simulink model "phdMain"  (R2023b)
settings: Solver=ode4  StartTime=0.0  StopTime=t.Data(end)  FixedStep=1e-3  RelTol=1e-3
undefined symbols (not defined in the file): A_bar, AEFF, B_E, C_bar, C_T, Cd_neg, Cd_pos, DiscIntNeverNeededParam, Gamma, H, k, K, L_gain, L_STROKE, M, m3PsToLpm, P_return_Pa, P_supply_Pa, PA_Pa, PaToBar, PB_Pa, Q, R, RHO, Ts, V01, V02, V_DEAD, v_mPs, W, xc_dot, xc_m
libraries: simulink x1
(part 2 of 3)

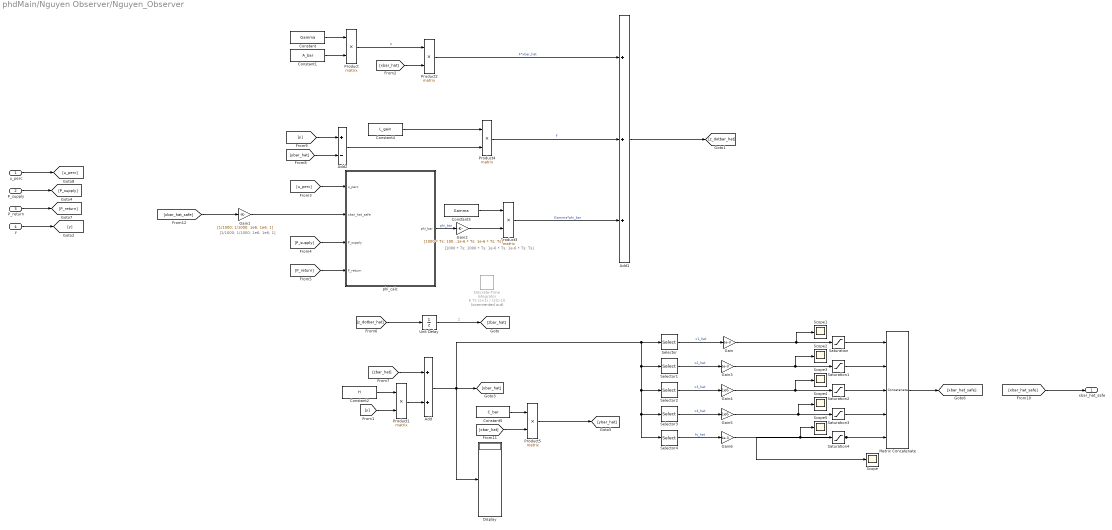
== system phdMain/Nguyen Observer/Nguyen_Observer ==
  note: [1000 * Ts; 1000 * Ts; 1e-6 * Ts; 1e-6 * Ts; Ts]
  note: [1/1000; 1/1000; 1e6; 1e6; 1]
  u_perc : Inport  PortDimensions=[1,1]
  P_supply : Inport  Port=2  OutDataTypeStr=double
  P_return : Inport  Port=3  OutDataTypeStr=double
  y : Inport  Port=4  PortDimensions=[4,1]
  Add : Sum
  Add1 : Sum  Inputs=+++
  Add2 : Sum  Inputs=+-
  Constant : Constant  Value=Gamma
  Constant1 : Constant  Value=A_bar
  Constant2 : Constant  Value=H
  Constant3 : Constant  Value=Gamma
  Constant4 : Constant  Value=L_gain
  Constant5 : Constant  Value=C_bar
  Discrete-Time Integrator : DiscreteIntegrator  Commented=on  IntegratorMethod=Integration: Trapezoidal  InitialCondition=[0,0,PA_Pa.Data(1)*1e-6,PB_Pa.Data(1)*1e-6,0]'  SampleTime=-1  ICPrevOutput=DiscIntNeverNeededParam  ICPrevScaledInput=DiscIntNeverNeededParam
  Display : Display
  Gain : Gain  Gain=1e-3
  Gain1 : Gain  Gain=[1/1000; 1/1000; 1e6; 1e6; 1]
  Gain2 : Gain  Gain=[1000 * Ts; 1000 * Ts; 1e-6 * Ts; 1e-6 * Ts; Ts]
  Gain3 : Gain  Gain=1e-3
  Gain4 : Gain  Gain=1e6
  Gain5 : Gain  Gain=1e6
  Gain6 : Gain  Gain=1e-3
  Matrix Concatenate : Concatenate  NumInputs=5  Mode=Multidimensional array
  Product{,1..5} (6 alike) : Product  Multiplication=Matrix(*)
  Saturation : Saturate  UpperLimit=L_STROKE  LowerLimit=-L_STROKE
  Saturation1 : Saturate  UpperLimit=2  LowerLimit=-2
  Saturation2 : Saturate  UpperLimit=200e5  LowerLimit=4e5
  Saturation3 : Saturate  UpperLimit=200e5  LowerLimit=4e5
  Saturation4 : Saturate  UpperLimit=L_STROKE  LowerLimit=-L_STROKE
  Scope{,1..5} (6 alike) : Scope
  Selector : Selector  InputPortWidth=5  IndexOptions=Index vector (dialog)  Indices=1  OutputSizes=1
  Selector1 : Selector  InputPortWidth=5  IndexOptions=Index vector (dialog)  Indices=2  OutputSizes=1
  Selector2 : Selector  InputPortWidth=5  IndexOptions=Index vector (dialog)  Indices=3  OutputSizes=1
  Selector3 : Selector  InputPortWidth=5  IndexOptions=Index vector (dialog)  Indices=4  OutputSizes=1
  Selector4 : Selector  InputPortWidth=5  IndexOptions=Index vector (dialog)  Indices=5  OutputSizes=1
  Unit Delay : UnitDelay  InitialCondition=[0,0,PA_Pa.Data(1)*1e-6,PB_Pa.Data(1)*1e-6,0]'  SampleTime=Ts  HasFrameUpgradeWarning=on
  phi_calc : Subsystem
  xbar_hat_safe : Outport
  wires:
  [y] -> Add2/1
  Product3/1 -> Add1/3  "Gamma*phi_bar"
  [u_perc] -> phi_calc/1(u_perc)
  Add2/1 -> Product4/2
  u_perc/1 -> [u_perc]
  Constant3/1 -> Product3/1
  Unit Delay/1 -> [zbar_hat]  "z"
  [ybar_hat] -> Add2/2
  Constant2/1 -> Product1/1
  Product/1 -> Product2/1  "F"
  [P_return] -> phi_calc/4(P_return)
  Constant1/1 -> Product/2
  Product2/1 -> Add1/1  "F*xbar_hat"
  Constant/1 -> Product/1
  [xbar_hat] -> Product2/2
  P_return/1 -> [P_return]
  [y] -> Product1/2
  [zbar_hat] -> Add/1
  y/1 -> [y]
  Add1/1 -> [z_dotbar_hat]
  Product4/1 -> Add1/2  "F"
  Product1/1 -> Add/2
  P_supply/1 -> [P_supply]
  phi_calc/1(phi_bar) -> Gain2/1  "phi_bar"
  [P_supply] -> phi_calc/3(P_supply)
  [z_dotbar_hat] -> Unit Delay/1
  [xbar_hat_safe] -> xbar_hat_safe/1
  Constant5/1 -> Product5/1
  [xbar_hat] -> Product5/2
  Product5/1 -> [ybar_hat]
  Selector3/1 -> Gain5/1  "x4_hat"
  Selector2/1 -> Gain4/1  "x3_hat"
  Selector1/1 -> Gain3/1  "x2_hat"
  Saturation/1 -> Matrix Concatenate/1
  Saturation1/1 -> Matrix Concatenate/2
  Saturation2/1 -> Matrix Concatenate/3
  Saturation3/1 -> Matrix Concatenate/4
  Saturation4/1 -> Scope/1, Matrix Concatenate/5
  Matrix Concatenate/1 -> [xbar_hat_safe]
  Selector4/1 -> Gain6/1  "fs_hat"
  Selector/1 -> Gain/1  "x1_hat"
  Constant4/1 -> Product4/1
  Add/1 -> Selector3/1, Selector4/1, Selector2/1, Selector1/1, Selector/1, [xbar_hat], Display/1
  [xbar_hat_safe] -> Gain1/1
  Gain1/1 -> phi_calc/2(xbar_hat_safe)
  Gain2/1 -> Product3/2
  Gain/1 -> Scope1/1, Saturation/1
  Gain3/1 -> Scope2/1, Saturation1/1
  Gain4/1 -> Saturation2/1, Scope3/1
  Gain5/1 -> Saturation3/1, Scope4/1
  Gain6/1 -> Scope5/1, Saturation4/1

== system phdMain/Reference_Generator/Sine_Generator ==
  Amp_mm : Inport  OutDataTypeStr=double
  f_Hz : Inport  Port=2
  phi_deg : Inport  Port=3  OutDataTypeStr=double
  Add : Sum
  Clock : Clock
  Constant : Constant  Value=2
  Constant1 : Constant  Value=3.14159265359
  Constant2 : Constant  Value=3.14159265359
  Constant3 : Constant  Value=180
  Constant4 : Constant  Value=1e-3
  Math Reciprocal : Math  Operator=reciprocal  SignedPower=on
  Product : Product  Inputs=4
  Product{1..4} (4 alike) : Product
  Sin : Trigonometry
  r : Outport
  wires:
  Constant1/1 -> Product/2
  Constant/1 -> Product/1
  f_Hz/1 -> Product/3
  phi_deg/1 -> Product1/1
  Constant2/1 -> Product2/1
  Constant3/1 -> Math Reciprocal/1
  Math Reciprocal/1 -> Product2/2
  Product2/1 -> Product1/2
  Clock/1 -> Product/4
  Product/1 -> Sin/1
  Sin/1 -> Product3/2
  Product1/1 -> Add/2
  Product3/1 -> Add/1
  Add/1 -> r/1
  Amp_mm/1 -> Product4/2
  Product4/1 -> Product3/1
  Constant4/1 -> Product4/1

== system phdMain/Reverse_PressureModel/Q_returnleak ==
  Add : Sum  Inputs=+-
  Constant5 : Constant  Value=70e5
  Divide : Product  Inputs=*/
  From Workspace20 : FromWorkspace  VariableName=P_supply_Pa
  From Workspace21 : FromWorkspace  VariableName=P_return_Pa
  Gain2 : Gain  Gain=0.53
  Sqrt : Sqrt
  Out1 : Outport
  wires:
  Constant5/1 -> Divide/2
  From Workspace20/1 -> Add/1  "P_supply"
  From Workspace21/1 -> Add/2  "P_return"
  Gain2/1 -> Out1/1
  Add/1 -> Divide/1
  Sqrt/1 -> Gain2/1
  Divide/1 -> Sqrt/1

== system phdMain/Reverse_PressureModel1/Q_returnleak ==
  Add : Sum  Inputs=+-
  Constant5 : Constant  Value=70e5
  Divide : Product  Inputs=*/
  From Workspace20 : FromWorkspace  VariableName=P_supply_Pa
  From Workspace21 : FromWorkspace  VariableName=P_return_Pa
  Gain2 : Gain  Gain=0.53
  Sqrt : Sqrt
  Out1 : Outport
  wires:
  Divide/1 -> Sqrt/1
  Sqrt/1 -> Gain2/1
  Add/1 -> Divide/1
  Gain2/1 -> Out1/1
  From Workspace21/1 -> Add/2  "P_return"
  From Workspace20/1 -> Add/1  "P_supply"
  Constant5/1 -> Divide/2

== system phdMain/SDRE_OBS_SNR/Subsystem ==
  Constant3 : Constant  Value=[1 0 0 0;0 0 1 0; 0 0 0 1]
  Constant4 : Constant  Value=mean(P_return_Pa)
  Constant5 : Constant  Value=Q
  Constant6 : Constant  Value=mean(P_supply_Pa)
  Constant7 : Constant  Value=R
  Discrete Algebraic Riccati Eqn : Subsystem
  MATLAB Function : MATLAB Function  TreatAsAtomicUnit=on
  MATLAB Function1 : MATLAB Function  TreatAsAtomicUnit=on
  MATLAB Function2 : MATLAB Function  TreatAsAtomicUnit=on
  Terminator : Terminator
  wires:
  [x4_hat] -> MATLAB Function2/5(x4_hat)
  MATLAB Function2/1(Q1) -> MATLAB Function1/1(Q1_calc)
  [x3_hat] -> MATLAB Function2/4(x3_hat)
  MATLAB Function1/1(B_x) -> Discrete Algebraic Riccati Eqn/2(B_k)
  [x1_hat] -> MATLAB Function/1(x_1_hat)
  Constant4/1 -> MATLAB Function2/3(Pr)
  MATLAB Function2/3(QR) -> Terminator/1
  MATLAB Function2/2(Q2) -> MATLAB Function1/2(Q2_calc)
  ? -> MATLAB Function2/1(u)
  [x2_hat] -> MATLAB Function/2(x_2_hat)
  Constant6/1 -> MATLAB Function2/2(Ps)
  Constant3/1 -> Discrete Algebraic Riccati Eqn/4(H)
  [y] -> Discrete Algebraic Riccati Eqn/3(y)
  Constant7/1 -> Discrete Algebraic Riccati Eqn/6(R)
  Constant5/1 -> Discrete Algebraic Riccati Eqn/5(Q)
  MATLAB Function/1(A_x) -> Discrete Algebraic Riccati Eqn/1(A_k)

== system phdMain/Subsystem3/Subsystem ==
  y : Inport
  phi2_hat : Inport  Port=2
  d1_hat : Inport  Port=3
  l1 : Inport  Port=4
  eta : Inport  Port=5
  phi1_hat : Inport  Port=6
  Add : Sum  Inputs=+-
  Add1 : Sum
  Add2 : Sum
  Product : Product
  Product1 : Product
  phi1_hat_dot : Outport
  wires:
  eta/1 -> Product/2
  l1/1 -> Product/1
  phi1_hat/1 -> Add/2
  y/1 -> Add/1
  Product/1 -> Product1/1
  Add/1 -> Product1/2
  Product1/1 -> Add1/2
  d1_hat/1 -> Add1/1
  Add1/1 -> Add2/2
  phi2_hat/1 -> Add2/1
  Add2/1 -> phi1_hat_dot/1

== system phdMain/Subsystem3/Subsystem1 ==
  phi1_hat : Inport
  d2_hat : Inport  Port=2
  l2 : Inport  Port=3
  eta : Inport  Port=4
  y : Inport  Port=5
  x3 : Inport  Port=6
  x4 : Inport  Port=7
  phi2_hat : Inport  Port=8
  Add : Sum  Inputs=+-
  Add1 : Sum
  Add2 : Sum
  Add3 : Sum  Inputs=+++
  Constant : Constant  Value=AEFF
  Constant1 : Constant  Value=M
  Divide : Product  Inputs=*/  RndMeth=Zero  SaturateOnIntegerOverflow=on
  Gain : Gain  Gain=1/M
  Lugre_Model : Subsystem
  Product{,1,3..4} (4 alike) : Product
  Unary Minus1 : UnaryMinus
  phi2_hat_dot : Outport
  wires:
  Add2/1 -> phi2_hat_dot/1
  Add1/1 -> Add2/2
  d2_hat/1 -> Add1/1
  Product1/1 -> Add1/2
  Add/1 -> Product1/2
  Product/1 -> Product1/1
  y/1 -> Add/1
  phi1_hat/1 -> Add/2
  l2/1 -> Product/1
  eta/1 -> Product/2
  Divide/1 -> Product3/1, Unary Minus1/1  "a23"
  x3/1 -> Product3/2
  Unary Minus1/1 -> Product4/1  "a24"
  x4/1 -> Product4/2
  Product3/1 -> Add3/2
  Product4/1 -> Add3/3
  Add3/1 -> Add2/1
  phi2_hat/1 -> Lugre_Model/1(xc_dot)
  Gain/1 -> Add3/1
  Lugre_Model/1(F_friction) -> Gain/1  "F_friction"
  Constant/1 -> Divide/1
  Constant1/1 -> Divide/2

== system phdMain/Subsystem3/Subsystem3 ==
  phi2_hat : Inport
  gamma1 : Inport  Port=2
  phi1_hat : Inport  Port=3
  sigma1_hat : Inport  Port=4
  Add : Sum
  Add1 : Sum
  Product : Product
  Product1 : Product
  Unary Minus : UnaryMinus
  sigma1_hat_dot : Outport
  wires:
  sigma1_hat/1 -> Add/1
  Product/1 -> Add/2
  Add/1 -> Add1/2
  phi2_hat/1 -> Add1/1
  gamma1/1 -> Unary Minus/1, Product/2
  phi1_hat/1 -> Product/1
  Add1/1 -> Product1/1
  Unary Minus/1 -> Product1/2
  Product1/1 -> sigma1_hat_dot/1

== system phdMain/Subsystem3/Subsystem4 ==
  phi2_hat : Inport
  gamma2 : Inport  Port=2
  x3 : Inport  Port=3
  x4 : Inport  Port=4
  sigma2_hat : Inport  Port=5
  Add : Sum
  Add2 : Sum
  Add3 : Sum  Inputs=+++
  Constant : Constant  Value=AEFF
  Constant1 : Constant  Value=M
  Divide : Product  Inputs=*/  RndMeth=Zero  SaturateOnIntegerOverflow=on
  Gain : Gain  Gain=1/M
  Lugre_Model : Subsystem
  Product{,1,3..4} (4 alike) : Product
  Unary Minus : UnaryMinus
  Unary Minus1 : UnaryMinus
  sigma2_hat_dot : Outport
  wires:
  Product1/1 -> sigma2_hat_dot/1
  gamma2/1 -> Unary Minus/1, Product/2
  Product/1 -> Add/2
  sigma2_hat/1 -> Add/1
  Product3/1 -> Add3/2
  Product4/1 -> Add3/3
  x4/1 -> Product4/2
  phi2_hat/1 -> Product/1, Lugre_Model/1(xc_dot)
  Unary Minus1/1 -> Product4/1  "a24"
  x3/1 -> Product3/2
  Add3/1 -> Add2/1
  Gain/1 -> Add3/1
  Add/1 -> Add2/2
  Add2/1 -> Product1/1
  Unary Minus/1 -> Product1/2
  Lugre_Model/1(F_friction) -> Gain/1  "F_friction"
  Constant/1 -> Divide/1
  Divide/1 -> Product3/1, Unary Minus1/1  "a23"
  Constant1/1 -> Divide/2

== system phdMain/Subsystem3/Subsystem6 ==
  sigma1_hat : Inport
  gamma1 : Inport  Port=2
  phi1_hat : Inport  Port=3
  Add : Sum
  Product : Product
  d1_hat : Outport
  wires:
  sigma1_hat/1 -> Add/1
  gamma1/1 -> Product/1
  phi1_hat/1 -> Product/2
  Product/1 -> Add/2
  Add/1 -> d1_hat/1

== system phdMain/Subsystem3/Subsystem7 ==
  sigma2_hat : Inport
  gamma2 : Inport  Port=2
  phi2_hat : Inport  Port=3
  Add : Sum
  Product : Product
  d2_hat : Outport
  wires:
  gamma2/1 -> Product/1
  sigma2_hat/1 -> Add/1
  Product/1 -> Add/2
  Add/1 -> d2_hat/1
  phi2_hat/1 -> Product/2

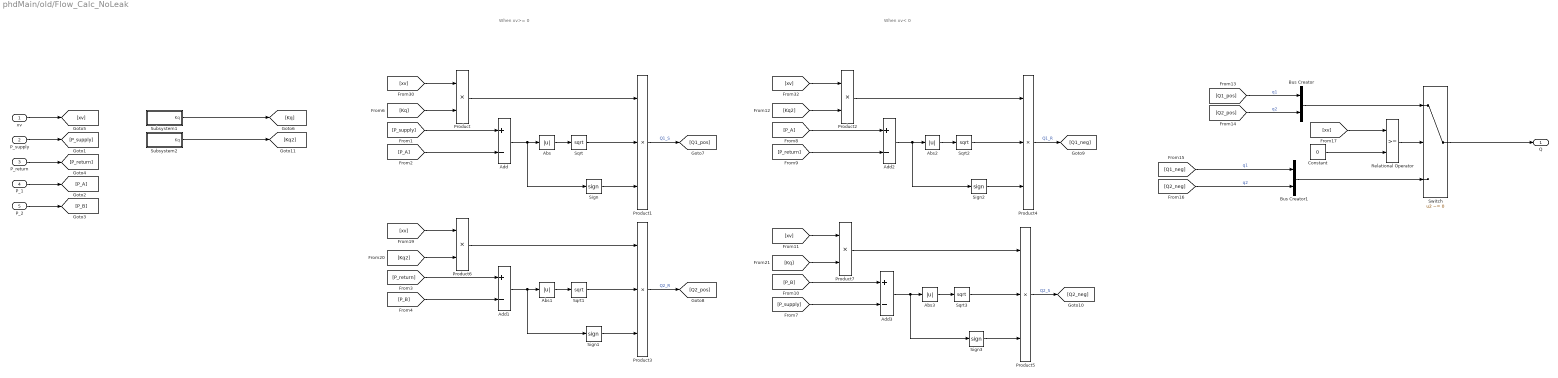
== system phdMain/old/Flow_Calc_NoLeak ==
  note: When xv< 0
  note: When xv>= 0
  xv : Inport  OutDataTypeStr=double
  P_supply : Inport  Port=2  OutDataTypeStr=double
  P_return : Inport  Port=3  OutDataTypeStr=double
  P_1 : Inport  Port=4  OutDataTypeStr=double
  P_2 : Inport  Port=5  OutDataTypeStr=double
  Abs{,1..3} (4 alike) : Abs  SaturateOnIntegerOverflow=off
  Add{,1..3} (4 alike) : Sum  Inputs=+-
  Bus Creator : BusCreator  Inputs=2
  Bus Creator1 : BusCreator  Inputs=2
  Constant : Constant  Value=0  OutDataTypeStr=double
  Product{,2,6..7} (4 alike) : Product
  Product{1,3..5} (4 alike) : Product  Inputs=3
  Relational Operator : RelationalOperator  OutDataTypeStr=boolean  RndMeth=Simplest  InputSameDT=off
  Sign{,1..3} (4 alike) : Signum
  Sqrt{,1..3} (4 alike) : Sqrt
  Subsystem1 : Subsystem
  Subsystem2 : Subsystem
  Switch : Switch  Criteria=u2 ~= 0  SaturateOnIntegerOverflow=off  InputSameDT=off
  Q : Outport  OutDataTypeStr=double
  wires:
  Subsystem2/1(Kq) -> [Kq2]
  Subsystem1/1(Kq) -> [Kq]
  Product5/1 -> [Q2_neg]  "Q2_S"
  Product4/1 -> [Q1_neg]  "Q1_R"
  Product3/1 -> [Q2_pos]  "Q2_R"
  Product1/1 -> [Q1_pos]  "Q1_S"
  Switch/1 -> Q/1
  [xv] -> Product/1
  [Q1_neg] -> Bus Creator1/1  "q1"
  [Q2_pos] -> Bus Creator/2  "q2"
  Product7/1 -> Product5/1
  [xv] -> Product7/1
  [Kq] -> Product7/2
  Product6/1 -> Product3/1
  [Kq2] -> Product6/2
  [xv] -> Product6/1
  Bus Creator1/1 -> Switch/3
  Bus Creator/1 -> Switch/1
  Relational Operator/1 -> Switch/2
  Constant/1 -> Relational Operator/2
  [xv] -> Relational Operator/1
  [Q2_neg] -> Bus Creator1/2  "q2"
  [Q1_pos] -> Bus Creator/1  "q1"
  [P_supply] -> Add3/2
  [P_B] -> Add3/1
  [P_return] -> Add2/2
  [P_A] -> Add2/1
  Product2/1 -> Product4/1
  Sqrt2/1 -> Product4/2
  Abs2/1 -> Sqrt2/1
  Add2/1 -> Abs2/1, Sign2/1
  Sign2/1 -> Product4/3
  Sign3/1 -> Product5/3
  Add3/1 -> Sign3/1, Abs3/1
  Abs3/1 -> Sqrt3/1
  Sqrt3/1 -> Product5/2
  [Kq2] -> Product2/2
  [xv] -> Product2/1
  xv/1 -> [xv]
  P_return/1 -> [P_return]
  P_2/1 -> [P_B]
  P_1/1 -> [P_A]
  P_supply/1 -> [P_supply]
  [P_B] -> Add1/2
  [P_return] -> Add1/1
  [Kq] -> Product/2
  Sqrt1/1 -> Product3/2
  Abs1/1 -> Sqrt1/1
  Add1/1 -> Abs1/1, Sign1/1
  Sign1/1 -> Product3/3
  Sign/1 -> Product1/3
  Add/1 -> Sign/1, Abs/1
  Abs/1 -> Sqrt/1
  Sqrt/1 -> Product1/2
  Product/1 -> Product1/1
  [P_A] -> Add/2
  [P_supply] -> Add/1

== system phdMain/old/Flow_Calc_WithLeak ==
  xv : Inport  OutDataTypeStr=double
  P_supply : Inport  Port=2  OutDataTypeStr=double
  P_return : Inport  Port=3  OutDataTypeStr=double
  P_1 : Inport  Port=4  OutDataTypeStr=double
  P_2 : Inport  Port=5  OutDataTypeStr=double
  Bus Creator4 : BusCreator  Inputs=2
  Constant1 : Constant  Value=RHO
  Constant19 : Constant  Value=3e-6
  Constant20 : Constant  Value=4e-6
  Constant22 : Constant  Value=0.6240657450358073
  Constant23 : Constant  Value=0.1382171870867411
  Constant24 : Constant  Value=0.7
  Constant26 : Constant  Value=82.43058647155762
  Constant27 : Constant  Value=W
  Constant28 : Constant  Value=0.01
  From Workspace2 : FromWorkspace  VariableName=[t.t, t.Q_return_m3Ps]
  Gain7 : Gain  Gain=m3PsToLpm
  Gain8 : Gain  Gain=1e-5
  Knob : KnobBlock  ScaleMin=0.1  ScaleMax=2
  Knob1 : KnobBlock  ScaleMin=0.1
  Knob2 : KnobBlock  ScaleMin=0.1  ScaleMax=2
  MATLAB Function2 : MATLAB Function  TreatAsAtomicUnit=on
  ReturnFlowDynamics1 : TransferFcn  Numerator=[28.61 633.5]  Denominator=[1 12.94 274.5 817.1]
  Scope : Scope  NumInputPorts=3
  q_withLeaks : Outport  OutDataTypeStr=double
  wires:
  P_supply/1 -> [P_supply]
  P_1/1 -> [P_A]
  P_2/1 -> [P_B]
  P_return/1 -> [P_return]
  xv/1 -> [xv]
  [xv] -> MATLAB Function2/1(xv)
  [P_supply] -> MATLAB Function2/2(P_P)
  [P_return] -> MATLAB Function2/3(P_T), MATLAB Function2/4(P_R)
  [P_A] -> MATLAB Function2/5(P_A)
  [P_B] -> MATLAB Function2/6(P_B)
  Constant27/1 -> MATLAB Function2/7(w)  "w"
  Constant19/1 -> MATLAB Function2/8(c)  "c"
  Constant20/1 -> MATLAB Function2/9(r)  "r"
  Constant1/1 -> MATLAB Function2/10(rho)  "rho"
  Constant28/1 -> MATLAB Function2/11(mu)  "mu"
  Constant24/1 -> MATLAB Function2/12(Cd)  "Cd"
  Constant22/1 -> MATLAB Function2/13(bias_P_dynamic)  "bias_P_dynamic"
  Constant23/1 -> MATLAB Function2/14(bias_T_dynamic)  "bias_T_dynamic"
  From Workspace2/1 -> Gain7/1
  Bus Creator4/1 -> q_withLeaks/1
  MATLAB Function2/1(Q_A) -> Bus Creator4/1  "q1"
  MATLAB Function2/2(Q_B) -> Bus Creator4/2  "q2"
  Constant26/1 -> Gain8/1  "x_leak"
  Gain8/1 -> MATLAB Function2/15(x_leak)
  MATLAB Function2/4(Q_return_model_lpm) -> [Q_return_model_lpm]
  MATLAB Function2/3(Q_Leak_Total_lpm) -> [Q_Leak_Total_lpm]
  Gain7/1 -> Scope/1  "Q_return_lpm"
  ReturnFlowDynamics1/1 -> Scope/3  "Q_returnTF_lpm"
  [Q_return_model_lpm] -> ReturnFlowDynamics1/1, Scope/2  "Q_return_model_lpm"

== system phdMain/old/ServoValve_Dynamics ==
  note: Deadband
  u : Inport  OutDataTypeStr=double
  Convert_SpoolPosition : Subsystem
  Dead Zone : DeadZone  LowerValue=-0.05  UpperValue=0.05
  Subsystem : Subsystem  Commented=on
  Valve Dynamics : TransferFcn  Numerator=[2.0884e+06]  Denominator=[1 2*1*1.4451e+03 2.0884e+06]
  xv : Outport  OutDataTypeStr=double
  wires:
  Dead Zone/1 -> Valve Dynamics/1
  u/1 -> Dead Zone/1
  Convert_SpoolPosition/1(xv) -> xv/1
  Valve Dynamics/1 -> Convert_SpoolPosition/1(u_perc)

== system phdMain/Cylinder_Dynamics/Lugre_Model/Subsystem1 ==
  term : Inport
  z_prev : Inport  Port=2
  v : Inport  Port=3
  Add : Sum
  Add1 : Sum
  Constant : Constant
  Gain : Gain  Gain=1e-3
  Gain1 : Gain  Gain=1e-3
  Math Reciprocal2 : Math  Operator=reciprocal  SignedPower=on
  Product : Product
  z : Outport
  wires:
  term/1 -> Gain1/1
  z_prev/1 -> Add/1
  v/1 -> Gain/1
  Gain/1 -> Add/2
  Add/1 -> Product/1
  Gain1/1 -> Add1/2
  Constant/1 -> Add1/1
  Add1/1 -> Math Reciprocal2/1
  Math Reciprocal2/1 -> Product/2
  Product/1 -> z/1

== system phdMain/Cylinder_Dynamics/Subsystem/Subsystem ==
  v_est : Inport
  MATLAB Function : MATLAB Function  TreatAsAtomicUnit=on
  F_statik : Outport
  wires:
  v_est/1 -> MATLAB Function/1(v)
  MATLAB Function/1(F_statik) -> F_statik/1

== system phdMain/Cylinder_Dynamics/Subsystem/Subsystem1 ==
  v_est : Inport
  MATLAB Function : MATLAB Function  TreatAsAtomicUnit=on
  F_statik : Outport
  wires:
  MATLAB Function/1(F_statik) -> F_statik/1
  v_est/1 -> MATLAB Function/1(v)

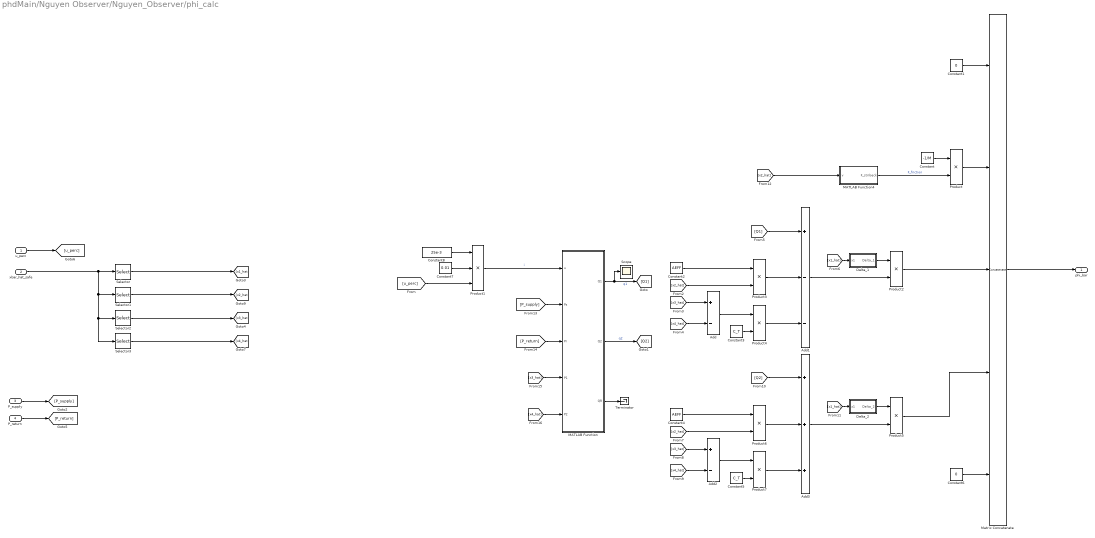
== system phdMain/Nguyen Observer/Nguyen_Observer/phi_calc ==
  u_perc : Inport
  xbar_hat_safe : Inport  Port=2
  P_supply : Inport  Port=3  OutDataTypeStr=double
  P_return : Inport  Port=4  OutDataTypeStr=double
  Add : Sum  Inputs=+-
  Add1 : Sum  Inputs=+--
  Add2 : Sum  Inputs=+-
  Add3 : Sum  Inputs=+++
  Constant : Constant  Value=-1/M
  Constant1 : Constant  Value=0
  Constant2 : Constant  Value=AEFF
  Constant3 : Constant  Value=C_T
  Constant4 : Constant  Value=AEFF
  Constant5 : Constant  Value=C_T
  Constant6 : Constant  Value=0
  Constant7 : Constant  Value=0.01
  Constant8 : Constant  Value=25e-3
  Delta_1 : Subsystem
  Delta_2 : Subsystem
  MATLAB Function : MATLAB Function  TreatAsAtomicUnit=on
  MATLAB Function4 : MATLAB Function  TreatAsAtomicUnit=on
  Matrix Concatenate : Concatenate  NumInputs=5  Mode=Multidimensional array
  Product{,2..7} (7 alike) : Product
  Product1 : Product  Inputs=3
  Scope : Scope
  Selector : Selector  InputPortWidth=5  IndexOptions=Index vector (dialog)  Indices=1  OutputSizes=1
  Selector1 : Selector  InputPortWidth=5  IndexOptions=Index vector (dialog)  Indices=2  OutputSizes=1
  Selector2 : Selector  InputPortWidth=5  IndexOptions=Index vector (dialog)  Indices=3  OutputSizes=1
  Selector3 : Selector  InputPortWidth=5  IndexOptions=Index vector (dialog)  Indices=4  OutputSizes=1
  Terminator : Terminator
  phi_bar : Outport
  wires:
  MATLAB Function4/1(F_stribeck) -> Product/2  "F_friction"
  Constant/1 -> Product/1
  MATLAB Function/1(Q1) -> Scope/1, [Q1]  "q1"
  MATLAB Function/2(Q2) -> [Q2]  "q2"
  [Q1] -> Add1/1
  [x2_hat] -> Product3/2
  [x4_hat] -> Add/2
  [x3_hat] -> Add/1
  Add/1 -> Product4/1
  Constant3/1 -> Product4/2
  Product3/1 -> Add1/2
  Product4/1 -> Add1/3
  Add1/1 -> Product2/2
  Delta_1/1(Delta_1) -> Product2/1
  [x1_hat] -> Delta_1/1(x1)
  [x1_hat] -> Delta_2/1(x1)
  Delta_2/1(Delta_2) -> Product5/1
  Add3/1 -> Product5/2
  Product7/1 -> Add3/3
  Product6/1 -> Add3/2
  Constant5/1 -> Product7/2
  Add2/1 -> Product7/1
  [x3_hat] -> Add2/1
  [x4_hat] -> Add2/2
  [x2_hat] -> Product6/2
  [Q2] -> Add3/1
  Constant6/1 -> Matrix Concatenate/5
  Product5/1 -> Matrix Concatenate/4
  Product/1 -> Matrix Concatenate/2
  Constant1/1 -> Matrix Concatenate/1
  Constant7/1 -> Product1/2
  Constant8/1 -> Product1/1
  Product1/1 -> MATLAB Function/1(u)  "i"
  u_perc/1 -> [u_perc]
  P_return/1 -> [P_return]
  P_supply/1 -> [P_supply]
  [u_perc] -> Product1/3
  [P_supply] -> MATLAB Function/2(Ps)
  [P_return] -> MATLAB Function/3(Pr)
  [x3_hat] -> MATLAB Function/4(P1)
  [x4_hat] -> MATLAB Function/5(P2)
  MATLAB Function/3(QR) -> Terminator/1
  Matrix Concatenate/1 -> phi_bar/1
  Selector/1 -> [x1_hat]
  Selector1/1 -> [x2_hat]
  Selector2/1 -> [x3_hat]
  Selector3/1 -> [x4_hat]
  Constant2/1 -> Product3/1
  Constant4/1 -> Product6/1
  Product2/1 -> Matrix Concatenate/3
  [x2_hat] -> MATLAB Function4/1(v)
  xbar_hat_safe/1 -> Selector3/1, Selector2/1, Selector1/1, Selector/1

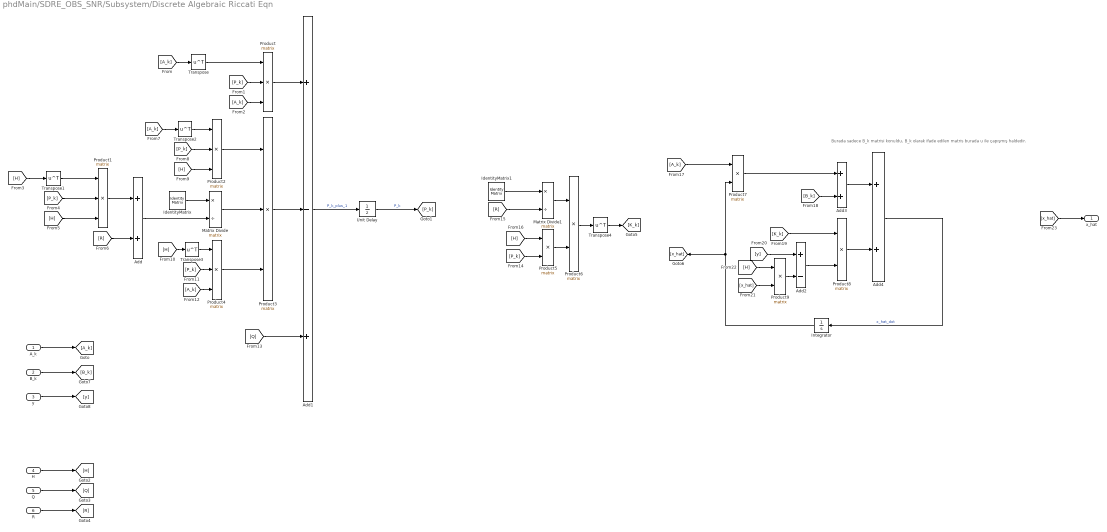
== system phdMain/SDRE_OBS_SNR/Subsystem/Discrete Algebraic Riccati Eqn ==
  note: Burada sadece B_k matrisi konuldu, B_k olarak ifade edilen matris burada u ile çapışmış haldedir.
  A_k : Inport  PortDimensions=[4,4]
  B_k : Inport  Port=2  PortDimensions=[4,1]
  y : Inport  Port=3
  H : Inport  Port=4
  Q : Inport  Port=5
  R : Inport  Port=6
  Add : Sum
  Add1 : Sum  Inputs=+-+
  Add2 : Sum  Inputs=+-
  Add3 : Sum
  Add4 : Sum
  IdentityMatrix : IdentityMatrix  OutputDimensions=4  SampleTime=1e-3
  IdentityMatrix1 : IdentityMatrix  OutputDimensions=3  SampleTime=1e-3
  Integrator : Integrator
  Matrix Divide : Product  Inputs=*/  Multiplication=Matrix(*)
  Matrix Divide1 : Product  Inputs=*/  Multiplication=Matrix(*)
  Product{,1..4} (5 alike) : Product  Inputs=3  Multiplication=Matrix(*)
  Product{5..9} (5 alike) : Product  Multiplication=Matrix(*)
  Transpose{,1..4} (5 alike) : Math  Operator=transpose
  Unit Delay : UnitDelay  SampleTime=-1  HasFrameUpgradeWarning=on
  x_hat : Outport
  wires:
  A_k/1 -> [A_k]
  [A_k] -> Transpose/1
  Transpose/1 -> Product/1
  [P_k] -> Product/2
  [A_k] -> Product/3
  H/1 -> [H]
  IdentityMatrix/1 -> Matrix Divide/1
  [H] -> Transpose1/1
  Transpose1/1 -> Product1/1
  [P_k] -> Product1/2
  [H] -> Product1/3
  Product1/1 -> Add/1
  [R] -> Add/2
  Add/1 -> Matrix Divide/2
  [A_k] -> Transpose2/1
  Transpose2/1 -> Product2/1
  [P_k] -> Product2/2
  [H] -> Product2/3
  Product2/1 -> Product3/1
  [P_k] -> Product4/2
  [H] -> Transpose3/1
  Transpose3/1 -> Product4/1
  [A_k] -> Product4/3
  Matrix Divide/1 -> Product3/2
  Product4/1 -> Product3/3
  Product/1 -> Add1/1
  Product3/1 -> Add1/2
  [Q] -> Add1/3
  Add1/1 -> Unit Delay/1  "P_k_plus_1"
  Unit Delay/1 -> [P_k]  "P_k"
  Q/1 -> [Q]
  R/1 -> [R]
  Matrix Divide1/1 -> Product6/1
  [R] -> Matrix Divide1/2
  IdentityMatrix1/1 -> Matrix Divide1/1
  [P_k] -> Product5/2
  [H] -> Product5/1
  Product5/1 -> Product6/2
  Product6/1 -> Transpose4/1
  Transpose4/1 -> [K_k]
  [A_k] -> Product7/1
  Integrator/1 -> [x_hat], Product7/2
  Product7/1 -> Add3/1
  [B_k] -> Add3/2
  B_k/1 -> [B_k]
  [K_k] -> Product8/1
  y/1 -> [y]
  [y] -> Add2/1
  Product9/1 -> Add2/2
  [x_hat] -> Product9/2
  [H] -> Product9/1
  Add2/1 -> Product8/2
  Product8/1 -> Add4/2
  Add3/1 -> Add4/1
  Add4/1 -> Integrator/1  "x_hat_dot"
  [x_hat] -> x_hat/1

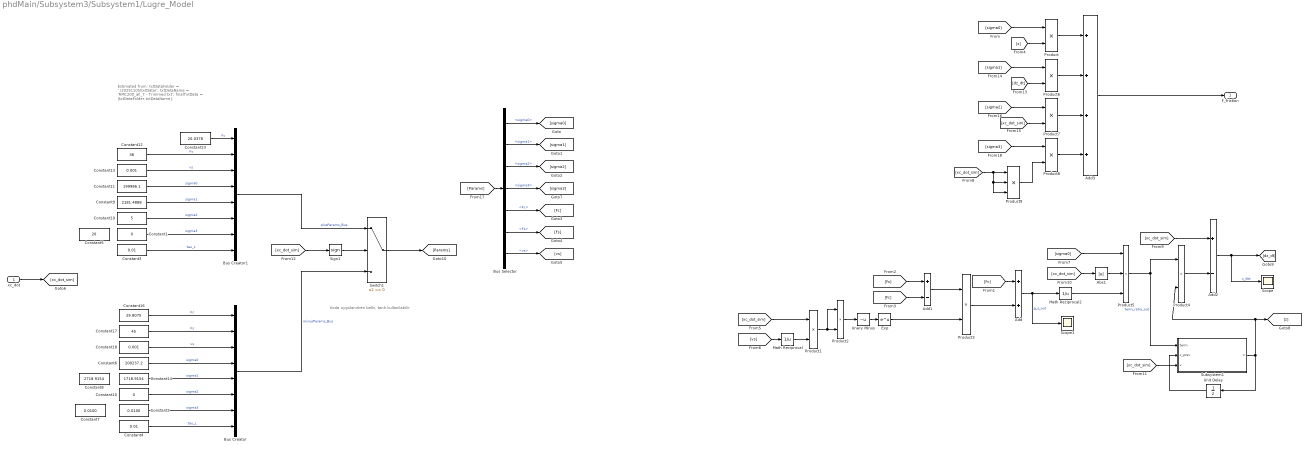
== system phdMain/Subsystem3/Subsystem1/Lugre_Model ==
  note: Koda uygulanırken belki, tanh kullanılabilir
  note: Estimated from:
      |
      | txtDataFolder = '.\20251105\txtData\';
      | txtDataName = 'RMC200_all_7 - Trimmed.txt';
      | finalTxtData = [txtDataFolder,txtDataName];
  xc_dot : Inport  OutDataTypeStr=double
  Abs1 : Abs  SaturateOnIntegerOverflow=off
  Add : Sum
  Add1 : Sum  Inputs=+-
  Add2 : Sum  Inputs=+-
  Add3 : Sum  Inputs=++++
  Bus Selector : BusSelector  OutputSignals=sigma0,sigma1,sigma2,sigma3,Fc,Fs,vs
  Bus Creator : BusCreator  Inputs=8
  Bus Creator1 : BusCreator  Inputs=8
  Constant1 : Constant  Value=0  OutDataTypeStr=double
  Constant10 : Constant  Value=0  OutDataTypeStr=double
  Constant11 : Constant  Value=199986.1  OutDataTypeStr=double
  Constant12 : Constant  Value=38  OutDataTypeStr=double
  Constant13 : Constant  Value=0.001  OutDataTypeStr=double
  Constant14 : Constant  Value=1718.9154  OutDataTypeStr=double
  Constant16 : Constant  Value=29.8075  OutDataTypeStr=double
  Constant17 : Constant  Value=45  OutDataTypeStr=double
  Constant18 : Constant  Value=0.001  OutDataTypeStr=double
  Constant19 : Constant  Value=5  OutDataTypeStr=double
  Constant2 : Constant  Value=0.0100  OutDataTypeStr=double
  Constant23 : Constant  Value=20.0378  OutDataTypeStr=double
  Constant3 : Constant  Value=0.01  OutDataTypeStr=double
  Constant4 : Constant  Value=0.01  OutDataTypeStr=double
  Constant5 : Constant  Value=20  OutDataTypeStr=double
  Constant6 : Constant  Value=200237.2  OutDataTypeStr=double
  Constant7 : Constant  Value=0.0100  OutDataTypeStr=double
  Constant8 : Constant  Value=2718.9154  OutDataTypeStr=double
  Constant9 : Constant  Value=2181.4888  OutDataTypeStr=double
  Exp : Math  SignedPower=on
  Math Reciprocal : Math  Operator=reciprocal  SignedPower=on
  Math Reciprocal2 : Math  Operator=reciprocal  SignedPower=on
  Product{,1..4,6..8} (8 alike) : Product
  Product5 : Product  Inputs=3
  Product9 : Product  Inputs=3
  Scope : Scope
  Scope1 : Scope
  Sign1 : Signum
  Subsystem1 : Subsystem
  Switch1 : Switch  SaturateOnIntegerOverflow=off  InputSameDT=off
  Unary Minus : UnaryMinus
  Unit Delay : UnitDelay  SampleTime=-1  HasFrameUpgradeWarning=on
  F_friction : Outport
  wires:
  Constant18/1 -> Bus Creator/3  "vs"
  Constant13/1 -> Bus Creator1/3  "vs"
  Constant12/1 -> Bus Creator1/2  "Fs"
  Constant17/1 -> Bus Creator/2  "Fs"
  Constant14/1 -> Bus Creator/5  "sigma1"
  Constant6/1 -> Bus Creator/4  "sigma0"
  Constant10/1 -> Bus Creator/6  "sigma2"
  Constant16/1 -> Bus Creator/1  "Fc"
  Constant9/1 -> Bus Creator1/5  "sigma1"
  Constant11/1 -> Bus Creator1/4  "sigma0"
  Constant19/1 -> Bus Creator1/6  "sigma2"
  Product7/1 -> Add3/3
  Product6/1 -> Add3/2
  [sigma2] -> Product7/1
  [xc_dot_sim] -> Product7/2
  [dz_dt] -> Product6/2
  [sigma1] -> Product6/1
  Product/1 -> Add3/1
  [z] -> Product/2
  [sigma0] -> Product5/1
  Abs1/1 -> Product5/2
  Add/1 -> Math Reciprocal2/1, Scope1/1  "g_s_out"
  [xc_dot_sim] -> Abs1/1
  Add1/1 -> Product3/1
  Unary Minus/1 -> Exp/1
  Product2/1 -> Unary Minus/1
  Product1/1 -> Product2/2, Product2/1
  [xc_dot_sim] -> Product1/1
  Math Reciprocal/1 -> Product1/2
  [vs] -> Math Reciprocal/1
  [Fc] -> Add1/2
  [Fs] -> Add1/1
  [Fc] -> Add/1
  [sigma0] -> Product/1
  Product3/1 -> Add/2
  [xc_dot_sim] -> Sign1/1
  Bus Creator1/1 -> Switch1/1  "plusParams_Bus"
  Bus Creator/1 -> Switch1/3  "minusParams_Bus"
  Switch1/1 -> [Params]
  [Params] -> Bus Selector/1
  Bus Selector/1 -> [sigma0]  "<sigma0>"
  Bus Selector/2 -> [sigma1]  "<sigma1>"
  Bus Selector/3 -> [sigma2]  "<sigma2>"
  Bus Selector/5 -> [Fc]  "<Fc>"
  Bus Selector/6 -> [Fs]  "<Fs>"
  Bus Selector/7 -> [vs]  "<vs>"
  Math Reciprocal2/1 -> Product5/3
  Exp/1 -> Product3/2
  Add2/1 -> Scope/1, [dz_dt]  "z_dot"
  Sign1/1 -> Switch1/2
  [xc_dot_sim] -> Add2/1
  Subsystem1/1(z) -> Product4/2, [z], Unit Delay/1
  [xc_dot_sim] -> Subsystem1/3(v)
  Unit Delay/1 -> Subsystem1/2(z_prev)
  Product5/1 -> Subsystem1/1(term), Product4/1  "term_ratio_out"
  Product4/1 -> Add2/2
  Add3/1 -> F_friction/1
  Constant1/1 -> Bus Creator1/7  "sigma3"
  Constant2/1 -> Bus Creator/7  "sigma3"
  Constant3/1 -> Bus Creator1/8  "tau_L"
  Constant4/1 -> Bus Creator/8  "tau_L"
  [sigma3] -> Product8/1
  Product8/1 -> Add3/4
  [xc_dot_sim] -> Product9/2, Product9/3, Product9/1
  Product9/1 -> Product8/2
  Bus Selector/4 -> [sigma3]  "<sigma3>"
  xc_dot/1 -> [xc_dot_sim]
  Constant23/1 -> Bus Creator1/1  "Fc"

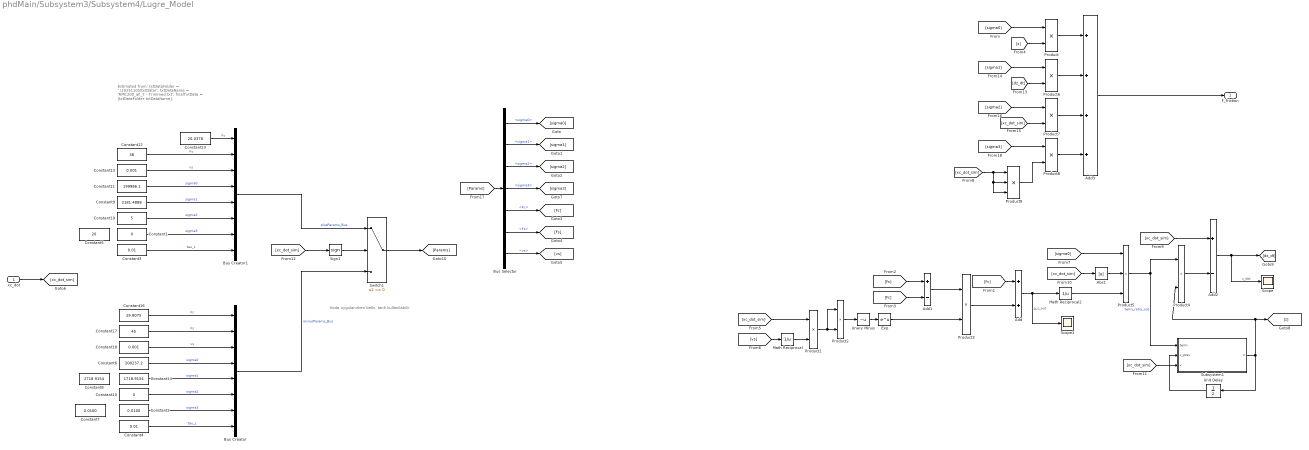
== system phdMain/Subsystem3/Subsystem4/Lugre_Model ==
  note: Koda uygulanırken belki, tanh kullanılabilir
  note: Estimated from:
      |
      | txtDataFolder = '.\20251105\txtData\';
      | txtDataName = 'RMC200_all_7 - Trimmed.txt';
      | finalTxtData = [txtDataFolder,txtDataName];
  xc_dot : Inport  OutDataTypeStr=double
  Abs1 : Abs  SaturateOnIntegerOverflow=off
  Add : Sum
  Add1 : Sum  Inputs=+-
  Add2 : Sum  Inputs=+-
  Add3 : Sum  Inputs=++++
  Bus Selector : BusSelector  OutputSignals=sigma0,sigma1,sigma2,sigma3,Fc,Fs,vs
  Bus Creator : BusCreator  Inputs=8
  Bus Creator1 : BusCreator  Inputs=8
  Constant1 : Constant  Value=0  OutDataTypeStr=double
  Constant10 : Constant  Value=0  OutDataTypeStr=double
  Constant11 : Constant  Value=199986.1  OutDataTypeStr=double
  Constant12 : Constant  Value=38  OutDataTypeStr=double
  Constant13 : Constant  Value=0.001  OutDataTypeStr=double
  Constant14 : Constant  Value=1718.9154  OutDataTypeStr=double
  Constant16 : Constant  Value=29.8075  OutDataTypeStr=double
  Constant17 : Constant  Value=45  OutDataTypeStr=double
  Constant18 : Constant  Value=0.001  OutDataTypeStr=double
  Constant19 : Constant  Value=5  OutDataTypeStr=double
  Constant2 : Constant  Value=0.0100  OutDataTypeStr=double
  Constant23 : Constant  Value=20.0378  OutDataTypeStr=double
  Constant3 : Constant  Value=0.01  OutDataTypeStr=double
  Constant4 : Constant  Value=0.01  OutDataTypeStr=double
  Constant5 : Constant  Value=20  OutDataTypeStr=double
  Constant6 : Constant  Value=200237.2  OutDataTypeStr=double
  Constant7 : Constant  Value=0.0100  OutDataTypeStr=double
  Constant8 : Constant  Value=2718.9154  OutDataTypeStr=double
  Constant9 : Constant  Value=2181.4888  OutDataTypeStr=double
  Exp : Math  SignedPower=on
  Math Reciprocal : Math  Operator=reciprocal  SignedPower=on
  Math Reciprocal2 : Math  Operator=reciprocal  SignedPower=on
  Product{,1..4,6..8} (8 alike) : Product
  Product5 : Product  Inputs=3
  Product9 : Product  Inputs=3
  Scope : Scope
  Scope1 : Scope
  Sign1 : Signum
  Subsystem1 : Subsystem
  Switch1 : Switch  SaturateOnIntegerOverflow=off  InputSameDT=off
  Unary Minus : UnaryMinus
  Unit Delay : UnitDelay  SampleTime=-1  HasFrameUpgradeWarning=on
  F_friction : Outport
  wires:
  Constant18/1 -> Bus Creator/3  "vs"
  Constant13/1 -> Bus Creator1/3  "vs"
  Constant12/1 -> Bus Creator1/2  "Fs"
  Constant17/1 -> Bus Creator/2  "Fs"
  Constant14/1 -> Bus Creator/5  "sigma1"
  Constant6/1 -> Bus Creator/4  "sigma0"
  Constant10/1 -> Bus Creator/6  "sigma2"
  Constant16/1 -> Bus Creator/1  "Fc"
  Constant9/1 -> Bus Creator1/5  "sigma1"
  Constant11/1 -> Bus Creator1/4  "sigma0"
  Constant19/1 -> Bus Creator1/6  "sigma2"
  Product7/1 -> Add3/3
  Product6/1 -> Add3/2
  [sigma2] -> Product7/1
  [xc_dot_sim] -> Product7/2
  [dz_dt] -> Product6/2
  [sigma1] -> Product6/1
  Product/1 -> Add3/1
  [z] -> Product/2
  [sigma0] -> Product5/1
  Abs1/1 -> Product5/2
  Add/1 -> Math Reciprocal2/1, Scope1/1  "g_s_out"
  [xc_dot_sim] -> Abs1/1
  Add1/1 -> Product3/1
  Unary Minus/1 -> Exp/1
  Product2/1 -> Unary Minus/1
  Product1/1 -> Product2/2, Product2/1
  [xc_dot_sim] -> Product1/1
  Math Reciprocal/1 -> Product1/2
  [vs] -> Math Reciprocal/1
  [Fc] -> Add1/2
  [Fs] -> Add1/1
  [Fc] -> Add/1
  [sigma0] -> Product/1
  Product3/1 -> Add/2
  [xc_dot_sim] -> Sign1/1
  Bus Creator1/1 -> Switch1/1  "plusParams_Bus"
  Bus Creator/1 -> Switch1/3  "minusParams_Bus"
  Switch1/1 -> [Params]
  [Params] -> Bus Selector/1
  Bus Selector/1 -> [sigma0]  "<sigma0>"
  Bus Selector/2 -> [sigma1]  "<sigma1>"
  Bus Selector/3 -> [sigma2]  "<sigma2>"
  Bus Selector/5 -> [Fc]  "<Fc>"
  Bus Selector/6 -> [Fs]  "<Fs>"
  Bus Selector/7 -> [vs]  "<vs>"
  Math Reciprocal2/1 -> Product5/3
  Exp/1 -> Product3/2
  Add2/1 -> Scope/1, [dz_dt]  "z_dot"
  Sign1/1 -> Switch1/2
  [xc_dot_sim] -> Add2/1
  Subsystem1/1(z) -> Product4/2, [z], Unit Delay/1
  [xc_dot_sim] -> Subsystem1/3(v)
  Unit Delay/1 -> Subsystem1/2(z_prev)
  Product5/1 -> Subsystem1/1(term), Product4/1  "term_ratio_out"
  Product4/1 -> Add2/2
  Add3/1 -> F_friction/1
  Constant1/1 -> Bus Creator1/7  "sigma3"
  Constant2/1 -> Bus Creator/7  "sigma3"
  Constant3/1 -> Bus Creator1/8  "tau_L"
  Constant4/1 -> Bus Creator/8  "tau_L"
  [sigma3] -> Product8/1
  Product8/1 -> Add3/4
  [xc_dot_sim] -> Product9/2, Product9/3, Product9/1
  Product9/1 -> Product8/2
  Bus Selector/4 -> [sigma3]  "<sigma3>"
  xc_dot/1 -> [xc_dot_sim]
  Constant23/1 -> Bus Creator1/1  "Fc"

== system phdMain/old/Flow_Calc_NoLeak/Subsystem1 ==
  Constant : Constant  Value=Cd_pos
  Constant1 : Constant  Value=W
  Constant2 : Constant  Value=RHO
  Constant3 : Constant  Value=2
  Math Reciprocal : Math  Operator=reciprocal  SignedPower=on
  Product : Product  Inputs=3
  Product1 : Product
  Sqrt : Sqrt
  Kq : Outport
  wires:
  Product/1 -> Kq/1
  Sqrt/1 -> Product/3
  Product1/1 -> Sqrt/1
  Constant3/1 -> Product1/1
  Math Reciprocal/1 -> Product1/2
  Constant2/1 -> Math Reciprocal/1  "rho"
  Constant1/1 -> Product/2  "w"
  Constant/1 -> Product/1  "Cd"

== system phdMain/old/Flow_Calc_NoLeak/Subsystem2 ==
  Constant : Constant  Value=Cd_neg
  Constant1 : Constant  Value=W
  Constant2 : Constant  Value=RHO
  Constant3 : Constant  Value=2
  Math Reciprocal : Math  Operator=reciprocal  SignedPower=on
  Product : Product  Inputs=3
  Product1 : Product
  Sqrt : Sqrt
  Kq : Outport
  wires:
  Constant/1 -> Product/1  "Cd"
  Constant1/1 -> Product/2  "w"
  Constant2/1 -> Math Reciprocal/1  "rho"
  Math Reciprocal/1 -> Product1/2
  Constant3/1 -> Product1/1
  Product1/1 -> Sqrt/1
  Sqrt/1 -> Product/3
  Product/1 -> Kq/1

== system phdMain/old/ServoValve_Dynamics/Convert_SpoolPosition ==
  u_perc : Inport  OutDataTypeStr=double
  Constant : Constant  Value=50e-3
  Constant1 : Constant  Value=0.01
  Constant2 : Constant  Value=0.001016
  Constant3 : Constant  Value=50e-3
  Math Reciprocal : Math  Operator=reciprocal  SignedPower=on
  Product : Product  Inputs=3
  Product1 : Product
  Product2 : Product
  xv : Outport  OutDataTypeStr=double
  wires:
  u_perc/1 -> Product/3
  Constant1/1 -> Product/2
  Constant3/1 -> Product/1
  Constant2/1 -> Product1/1
  Math Reciprocal/1 -> Product1/2
  Constant/1 -> Math Reciprocal/1
  Product1/1 -> Product2/2  "Ki"
  Product/1 -> Product2/1  "i"
  Product2/1 -> xv/1  "xv"

== system phdMain/old/ServoValve_Dynamics/Subsystem ==
  Valve Dynamics1 : TransferFcn  Numerator=[7.738e05]  Denominator=[1 1244 7.738e05]
  Valve Dynamics2 : TransferFcn  Numerator=[(120*2*pi)^2]  Denominator=[1 2*0.95*(120*2*pi) (120*2*pi)^2]

== system phdMain/Nguyen Observer/Nguyen_Observer/phi_calc/Delta_1 ==
  x1 : Inport
  Add2 : Sum
  Constant5 : Constant  Value=B_E
  Constant6 : Constant  Value=AEFF
  Constant7 : Constant  Value=V01
  Gain : Gain  Gain=1e-2
  Math Reciprocal : Math  Operator=reciprocal  SignedPower=on
  Product5 : Product
  Product6 : Product
  Delta_1 : Outport
  wires:
  Product5/1 -> Add2/2
  Constant5/1 -> Gain/1
  Math Reciprocal/1 -> Product6/2
  x1/1 -> Product5/2
  Product6/1 -> Delta_1/1
  Add2/1 -> Math Reciprocal/1
  Constant6/1 -> Product5/1
  Constant7/1 -> Add2/1
  Gain/1 -> Product6/1

== system phdMain/Nguyen Observer/Nguyen_Observer/phi_calc/Delta_2 ==
  x1 : Inport
  Add2 : Sum  Inputs=+-
  Constant5 : Constant  Value=B_E
  Constant6 : Constant  Value=AEFF
  Constant7 : Constant  Value=V02
  Gain2 : Gain  Gain=1e-2
  Math Reciprocal : Math  Operator=reciprocal  SignedPower=on
  Product5 : Product
  Product6 : Product
  Delta_2 : Outport
  wires:
  Add2/1 -> Math Reciprocal/1
  Product6/1 -> Delta_2/1
  x1/1 -> Product5/2
  Math Reciprocal/1 -> Product6/2
  Constant5/1 -> Gain2/1
  Product5/1 -> Add2/2
  Constant6/1 -> Product5/1
  Constant7/1 -> Add2/1
  Gain2/1 -> Product6/1

== system phdMain/Subsystem3/Subsystem1/Lugre_Model/Subsystem1 ==
  term : Inport
  z_prev : Inport  Port=2
  v : Inport  Port=3
  Add : Sum
  Add1 : Sum
  Constant : Constant
  Gain : Gain  Gain=1e-3
  Gain1 : Gain  Gain=1e-3
  Math Reciprocal2 : Math  Operator=reciprocal  SignedPower=on
  Product : Product
  z : Outport
  wires:
  term/1 -> Gain1/1
  z_prev/1 -> Add/1
  v/1 -> Gain/1
  Gain/1 -> Add/2
  Add/1 -> Product/1
  Gain1/1 -> Add1/2
  Constant/1 -> Add1/1
  Add1/1 -> Math Reciprocal2/1
  Math Reciprocal2/1 -> Product/2
  Product/1 -> z/1

== system phdMain/Subsystem3/Subsystem4/Lugre_Model/Subsystem1 ==
  term : Inport
  z_prev : Inport  Port=2
  v : Inport  Port=3
  Add : Sum
  Add1 : Sum
  Constant : Constant
  Gain : Gain  Gain=1e-3
  Gain1 : Gain  Gain=1e-3
  Math Reciprocal2 : Math  Operator=reciprocal  SignedPower=on
  Product : Product
  z : Outport
  wires:
  term/1 -> Gain1/1
  z_prev/1 -> Add/1
  v/1 -> Gain/1
  Gain/1 -> Add/2
  Add/1 -> Product/1
  Gain1/1 -> Add1/2
  Constant/1 -> Add1/1
  Add1/1 -> Math Reciprocal2/1
  Math Reciprocal2/1 -> Product/2
  Product/1 -> z/1

== matlab function phdMain/Cylinder_Dynamics/MATLAB Function2 ==
  data: v input; FF output
function FF = fcn(v)
eps_smooth = 0.002; 

% --- Pozitif Yön (v > 0) ---
kv_p = 20; kc_p = 15; ks_p = 82.9; tau_p = 0.016;

% --- Negatif Yön (v < 0) ---
kv_n = 35; kc_n = 22; ks_n = 75.17; tau_n = 0.016;

% Yumuşatılmış yön fonksiyonu (sign yerine tanh)
% Bu fonksiyon -1 ile 1 arasında yumuşak bir geçiş sağlar
smooth_sign = tanh(v ./ eps_smooth);

% Asimetrik katsayı vektörleri oluşturma
% Hızın yönüne göre katsayıları seçiyoruz
kv = (v >= 0)*kv_p + (v < 0)*kv_n;
kc = (v >= 0)*kc_p + (v < 0)*kc_n;
ks = (v >= 0)*ks_p + (v < 0)*ks_n;
tau = (v >= 0)*tau_p + (v < 0)*tau_n;

% --- Sürtünme Kuvveti Hesaplama ---
% F_viscous + F_coulomb + F_stribeck
FF = (kv .* v) + (kc .* smooth_sign) + (ks .* smooth_sign .* exp(-abs(v./tau)));

== matlab function phdMain/Cylinder_Dynamics/Subsystem/Kalman_Jerk_xa ==
  settings: updateMethod=DISCRETE
  data: pos_meas input; v_est output; acc_meas input; dt input; a_est output; j_est output
function [v_est, a_est, j_est] = fcn(pos_meas, acc_meas, dt)
    % KALMAN FİLTRESİ (Jerk Augmented)
    % Durumlar: x = [Pozisyon; Hız; İvme; Jerk]
    
    % Değişkenleri hafızada tutmak için 'persistent' tanımlıyoruz
    persistent x P A H Q R I initialized
    
    % --- BAŞLANGIÇ AYARLARI (Sadece ilk adımda çalışır) ---
    if isempty(initialized)
        % Başlangıç Durumu (İlk ölçüme göre)
        x = [pos_meas; 0; acc_meas; 0]; 
        
        % Başlangıç Belirsizliği
        P = eye(4); 
        
        % Matris Tanımları (Sabitler)
        % 1. Geçiş Matrisi (Fizik: x = x0 + v*dt + 0.5*a*dt^2 + ...)
        A = [1, dt, 0.5*dt^2, (1/6)*dt^3;
             0,  1,       dt,   0.5*dt^2;
             0,  0,        1,         dt;
             0,  0,        0,          1];
         
        % 2. Ölçüm Matrisi (Sadece Pos ve Acc ölçüyoruz)
        H = [1, 0, 0, 0;
             0, 0, 1, 0];
         
        % 3. Gürültü Kovaryansları (TUNING BURADAN)
        sigma_jerk = 2000; % Sistemin vahşiliği (Spike yakalama yeteneği)
        
        % Q (Süreç Gürültüsü)
        Q = diag([dt^6/36, dt^4/4, dt^2, 1]) * sigma_jerk^2;
        
        % R (Ölçüm Gürültüsü) - Sensör güveni
        R_pos = (1e-6)^2;
        R_acc = (0.5)^2;
        R = diag([R_pos, R_acc]);
        
        I = eye(4);
        initialized = 1;
    end
    
    % --- KALMAN DÖNGÜSÜ (Her adımda çalışır) ---
    
    % 1. PREDICT (Öngörü)
    x_pred = A * x;
    P_pred = A * P * A' + Q;
    
    % 2. UPDATE (Düzeltme)
    z = [pos_meas; acc_meas]; % Ölçüm vektörü
    
    y = z - H * x_pred;       % Innovation (Hata)
    S = H * P_pred * H' + R;  % Innovation Covaryans
    K = P_pred * H' / S;      % Kalman Kazancı
    
    x = x_pred + K * y;       % Durum Güncelleme
    P = (I - K * H) * P_pred; % Kovaryans Güncelleme
    
    % 3. ÇIKTI
    v_est = x(2);
    a_est = x(3);
    j_est = x(4);
end

== matlab function phdMain/Cylinder_Dynamics/Subsystem/Kalman_Jerk_xPaPb ==
  settings: updateMethod=DISCRETE
  data: j_est output; a_est output; pos_meas input; v_est output; PA input; PB input
function [j_est, a_est, v_est] = fcn(pos_meas, PA, PB)
    % PRESSURE-AIDED JERK ESTIMATOR
    % Girdiler: Pozisyon ve Basınçlar
    % Çıktı: Tertemiz Jerk (j_est)
    
    persistent x P A H Q R I initialized m AA AB
    
    % --- SABİTLER ---
    dt = 0.001;   % Örnekleme Zamanı (Simulink step size ile aynı olmalı)
    
    if isempty(initialized)
        % 1. SİSTEM TANIMLAMALARI
        m  = 3.4;       % Tahmini Hareketli Kütle (kg)
        AA = 2.0106e-04;  % A Odası Alanı (m2)
        AB = 2.0106e-04;  % B Odası Alanı (m2)
        
        % 2. DURUM VEKTÖRÜ: x = [Konum; Hız; İvme; Jerk]
        % (Sürtünme değil, doğrudan kinematiği izliyoruz)
        F_net_start = (PA*AA - PB*AB);
        a_start = F_net_start / m;
        
        x = [pos_meas; 0; a_start; 0];
        P = eye(4);
        I = eye(4);
        
        % 3. GEÇİŞ MATRİSİ (Constant Jerk Model)
        % x(k+1) = x(k) + v*dt + 0.5*a*dt^2 + 1/6*j*dt^3 ...
        A = [1, dt, 0.5*dt^2, (1/6)*dt^3;
             0,  1,       dt,   0.5*dt^2;
             0,  0,        1,         dt;
             0,  0,        0,          1];
         
        % 4. ÖLÇÜM MATRİSİ
        % z1 = Konum (x1)
        % z2 = İvme  (x3) -> Basınçtan türetilmiş "Sanal İvme"
        H = [1, 0, 0, 0;
             0, 0, 1, 0];
         
        % 5. TUNING (AYARLAR)
        % Q: Jerk ne kadar hızlı değişebilir? (Sistemin vahşiliği)
        % Yüksek değer = Zıplamaları anında yakalar (Gecikmesiz).
        sigma_jerk = 100; 
        Q = diag([dt^6/36, dt^4/4, dt^2, 1]) * sigma_jerk^2;
        
        % R: Ölçümlere ne kadar güveniyoruz?
        R_pos = (1e-6)^2; % Konum çok hassas
        R_acc = (2.0)^2;  % Basınçtan gelen ivme "gürültülüdür" (Sürtünme yok sayıldığı için)
                          % Burayı gevşek bırakıyoruz ki Kalman, konum verisiyle
                          % basınç verisini harmanlayıp doğruyu bulsun.
        R = diag([R_pos, R_acc]);
        
        initialized = 1;
    end
    
    % --- 1. SANAL İVME ÖLÇÜMÜ OLUŞTURMA ---
    % Basınç kuvvetini kütleye bölerek "Ham İvme" elde ediyoruz.
    % Not: Bu ivme sürtünmeyi içermez, bu yüzden "gürültülü/hatalı" kabul edilir.
    % Kalman bunu düzeltecek.
    F_hyd = PA * AA - PB * AB;
    a_meas_virtual = F_hyd / m; 
    
    % Ölçüm Vektörü
    z = [pos_meas; a_meas_virtual];
    
    % --- 2. KALMAN PREDICT ---
    x_pred = A * x;
    P_pred = A * P * A' + Q;
    
    % --- 3. KALMAN UPDATE ---
    y = z - H * x_pred;       % Hata (Innovation)
    S = H * P_pred * H' + R;  % Kovaryans
    K = P_pred * H' / S;      % Kazanç (Gain)
    
    x = x_pred + K * y;       % Güncelleme
    P = (I - K * H) * P_pred;
    
    % --- 4. ÇIKTILAR ---
    v_est = x(2);
    a_est = x(3);
    j_est = x(4); % İŞTE ARADIĞIN JERK!
end

== matlab function phdMain/Cylinder_Dynamics/Subsystem/Subsystem1/MATLAB Function ==
  data: v input; F_statik output
function F_statik = fcn(v)
Fc = 18; 
Fs = 75; 
v_s = 0.016; 
C = 100; 

F_statik = Fc + (Fs - Fc)*exp(-(1*abs(v)./v_s)^2);
F_statik = F_statik * tanh(C*v);

== matlab function phdMain/Cylinder_Dynamics/MATLAB Function1 ==
  data: v input; FF output; a input; j input
function FF = fcn(v,a,j)
% --- Geçiş Yumuşaklığı Parametresi ---
% Bu değer büyüdükçe 0'daki eğim azalır (daha eğimli geçer)
eps_smooth = 0.00223;


% --- Pozitif Yön (v > 0) ---
kv_p = 39.658; Fc_p = 25; Fs_p = 82.9; tau_p = 0.0016;

% --- Negatif Yön (v < 0) ---
kv_n = 38.5; Fc_n = 5; Fs_n = 75.17; tau_n = 0.0016;

% Yumuşatılmış yön fonksiyonu (sign yerine tanh)
% Bu fonksiyon -1 ile 1 arasında yumuşak bir geçiş sağlar
smooth_sign = tanh(v ./ eps_smooth);

% Asimetrik katsayı vektörleri oluşturma
% Hızın yönüne göre katsayıları seçiyoruz
kv = (v >= 0)*kv_p + (v < 0)*kv_n;
Fc = (v >= 0)*Fc_p + (v < 0)*Fc_n;
Fs = (v >= 0)*Fs_p + (v < 0)*Fs_n;
tau = (v >= 0)*tau_p + (v < 0)*tau_n;

F_stribeck = (kv .* v) + (Fc .* smooth_sign) + (Fs .* smooth_sign .* exp(-abs(v./tau)));

K_acc = 1.121235; 
K_jerk = 0.056481; 
kappa_delay = 0; 

FF = F_stribeck + K_acc * a  +  K_jerk*j;

== matlab function phdMain/Cylinder_Dynamics/MATLAB Function3 ==
  data: v input; F_friction_nodelay output; FF input; j input; a input
function F_friction_nodelay = fcn(v, FF, j, a)

K_acc_p = 1.021235; 
K_acc_n = 0.0810121235; 

K_jerk_p = -0.05656481; 
K_jerk_n = 0.02056481; 

K_acc = (v>=0)*K_acc_p + (v<0)*K_acc_n; 
K_jerk = (v>=0)*K_jerk_p + (v<0)*K_jerk_n; 

F_friction_nodelay = FF + K_acc .* a  +  K_jerk.*j;

== matlab function phdMain/Cylinder_Dynamics/MATLAB Function4 ==
  data: v input; F_stribeck output
function F_stribeck = fcn(v)


% close all 

% --- Geçiş Yumuşaklığı Parametresi ---
% Bu değer büyüdükçe 0'daki eğim azalır (daha eğimli geçer)
eps_smooth = 0.0223;
% eps_smooth = 0.015;

%%%
kv_p = 12; Fc_p = 25; Fs_p  = 383; tau_p = 0.016;
kv_n = 35; Fc_n = 7.5; Fs_n = 183; tau_n = 0.02016;
%%%


% Yumuşatılmış yön fonksiyonu (sign yerine tanh)
% Bu fonksiyon -1 ile 1 arasında yumuşak bir geçiş sağlar
smooth_sign = tanh(v ./ eps_smooth);

% Asimetrik katsayı vektörleri oluşturma
% Hızın yönüne göre katsayıları seçiyoruz
kv = (v >= 0)*kv_p + (v < 0)*kv_n;
Fc = (v >= 0)*Fc_p + (v < 0)*Fc_n;
Fs = (v >= 0)*Fs_p + (v < 0)*Fs_n;
tau = (v >= 0)*tau_p + (v < 0)*tau_n;
F_stribeck = (kv .* v) + (Fc .* smooth_sign) + (Fs .* smooth_sign .* exp(-abs(v./tau)));

== matlab function phdMain/Nguyen Observer/Nguyen_Observer/phi_calc/MATLAB Function ==
  data: Q1 output; Q2 output; u input; Ps input; Pr input; P1 input; P2 input; QR output
function [Q1, Q2, QR] = fcn(u, Ps, Pr, P1, P2)
    % x0 parametresini girişten kaldırdık, içeride asimetrik tanımlayacağız.
    % Valve params 
    K           = 0.00000334; 
    k           = 1.82709080; 

    % --- ASİMETRİK SIZINTI AYARLARI ---
    % Hedef: P_null = 70 bar (Ps=210 bar iken)
    % Bu dengeyi sağlamak için Return tarafı açıklığı daha büyük olmalı.

    % --- GÜNCELLENMİŞ ASİMETRİK SIZINTI AYARLARI ---
    % Hedef: Ps=200 bar, Pr=4.5 bar iken yaklaşık 70-75 bar denge basıncı
    % $$x_{0S} \cdot \sqrt{130} = x_{0R} \cdot \sqrt{70}$$ --> Ortalamaları
    % da bulunan x0 olacak.

    % Ortalama x0 = 0.53e-3 idi. Bunu asimetrik dağıtıyoruz:
    % x0_S = 0.47e-3;  % Supply tarafı (0.47 mA)
    % x0_R = 0.64e-3;  % Return tarafı (0.64 mA)
    
    x0_S = 0.46e-3 ;  % Supply tarafı (0.46 mA) --> bunu editledim
    x0_R = 0.64e-3 ;  % Return tarafı (0.64 mA)

    % x0_S = 0.53e-3;  % Supply tarafı (0.47 mA)
    % x0_R = 0.53e-3;  % Return tarafı (0.64 mA)

    K_tare = 2.345e-9; 
    
    % Güvenlik (Basınçlar)
    dPs1 = max(0, Ps - P1); dP1r = max(0, P1 - Pr);
    dPs2 = max(0, Ps - P2); dP2r = max(0, P2 - Pr);
    dPsr = max(0, Ps - Pr);

    if u >= 0
        % P_S -> P_1 (Supply Side - Ana Akış) -> x0_S kullan
        Q1_S = K * sqrt(dPs1) * (x0_S + u); 
        
        % P_1 -> P_R (Return Side - Sızıntı) -> x0_R kullan
        Q1_R = K * sqrt(dP1r) * (x0_R^2 / (x0_R + k*u)); 

        % P_S -> P_2 (Supply Side - Sızıntı) -> x0_S kullan
        Q2_S = K * sqrt(dPs2) * (x0_S^2 / (x0_S + k*u)); 
        
        % P_2 -> P_R (Return Side - Ana Akış) -> x0_R kullan
        Q2_R = K * sqrt(dP2r) * (x0_R + u);
    else
        % x < 0 durumu
        % Simetriyi korumak için x negatifken de Supply/Return rollerine göre
        % doğru x0'ı seçmeliyiz.
        
        % P_S -> P_1 (Supply Side - Sızıntı)
        Q1_S = K * sqrt(dPs1) * (x0_S^2 / (x0_S - k*u)); 
        
        % P_1 -> P_R (Return Side - Ana Akış)
        Q1_R = K * sqrt(dP1r) * (x0_R - u); 

        % P_S -> P_2 (Supply Side - Ana Akış)
        Q2_S = K * sqrt(dPs2) * (x0_S - u); 
        
        % P_2 -> P_R (Return Side - Sızıntı)
        Q2_R = K * sqrt(dP2r) * (x0_R^2 / (x0_R - k*u)); 
    end

    Q1 = Q1_S - Q1_R;
    Q2 = Q2_S - Q2_R;
    QR = Q1_R + (Q2_R) + K_tare * sqrt(dPsr); 
end

== matlab function phdMain/SDRE_OBS_SNR/Subsystem/MATLAB Function ==
  data: x_1_hat input; A_x output; x_2_hat input
function A_x = A_x(x_1_hat, x_2_hat)

M           = 3.4;                      % Movable mass (Piston + Rod) kg
D_PISTON    = 34e-3;                    % Piston Diameter m
D_ROD       = 30e-3;                    % Rod Diameter m
A_PISTON    = (pi * D_PISTON^2)/4;      % Piston area m^2
A_ROD       = (pi * D_ROD^2)/4;         % Rod area m^2
AEFF        = A_PISTON - A_ROD;         % Effective Area m2
L_STROKE    = 190.16e-3;                % Total Stroke Length m
V01         = AEFF * (L_STROKE/2);      % Initial Chamber Volume in neural position m^3
V02         = AEFF * (L_STROKE/2);      % Initial Chamber Volume in neural position m^3
V_DEAD      = 1.5315e-05;               % 15.3 cm^3 dead volume <- 
V0 = V01 + V_DEAD;                      % Total Volume m3
C_T = 3.9933e-13;                       % Internal leakage constant m3/s/Pa
B_V = 28.08;                            % Viskoz sürtünme katsayısı N.s/m
F_s = 88.30;                            % Statik sürtünme değeri N 
F_c = 16.63;                            % Coulomb sürtünme değeri N 
tau = 0.03695;                          % Stribeck velocity coefficient 

eps = 1e-6;                             % Epsilon for numerical stability 
%%
m = M; 
B = B_V;
C_t = C_T; 
A_c = AEFF; 
V_0 = V0; 
beta = 1.6e9; 

%%
if x_2 >=0 
    F_c = 6.93; 
    F_s = 93.02; 
    tau = 0.0357; 
    B = 33.96; 
else 
    F_c = 19.39; 
    F_s = 83.58; 
    tau = 0.0382; 
    B = 31.98; 
end 
F_frc = tanh(x_2) * (F_c + (F_s-F_c)*exp(-(abs(x_2))/(tau))); % sürtünme denkleminde sign yerine tanh kullanıldı


delta_1 = beta / ((V_0 + A_c*x_1_hat));
delta_2 = beta / ((V_0 - A_c*x_1_hat));

a22 = -B/m - F_frc/(m*abs(x_2_hat) + eps);
a23 = A_c/m;
a24 = -A_c/m;
a32 = -delta_1*A_c; 
a33 = -delta_1*C_t;
a34 = delta_1*C_t;
a42 = delta_2*A_c;
a43 = delta_2*C_t;
a44 = -delta_2*C_t;


A_x = [0    1       0       0; 
       0    a22     a23     a24; 
       0    a32     a33     a34; 
       0    a42     a43     a44];
end
